simulink model "sistema_circuito2"  (R2025a)
settings: Solver=ode23tb  StartTime=0.0  StopTime=10.0  MaxStep=1E-3  RelTol=1e-3
libraries: fl_lib x12, ee_lib x3, nesl_utility x3
settings Model: Creator=Abigail VC  LastModifiedBy=Abigail VC
settings DataIOCC: TimeSaveName=t
settings DebuggingCC: AlgebraicLoopMsg=none  ArtificialAlgebraicLoopMsg=none  MaxConsecutiveZCsMsg=none

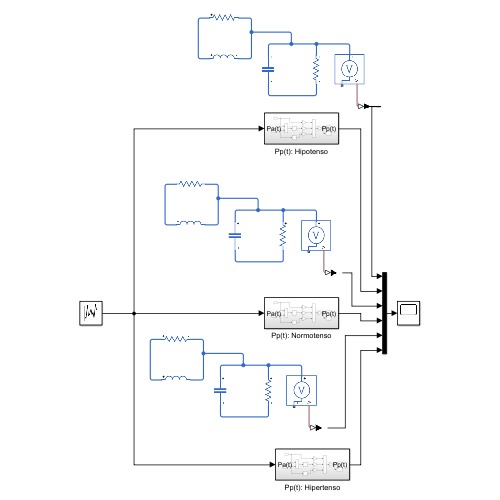
[thumbnail: Simulink's stored preview of the top-level diagram]
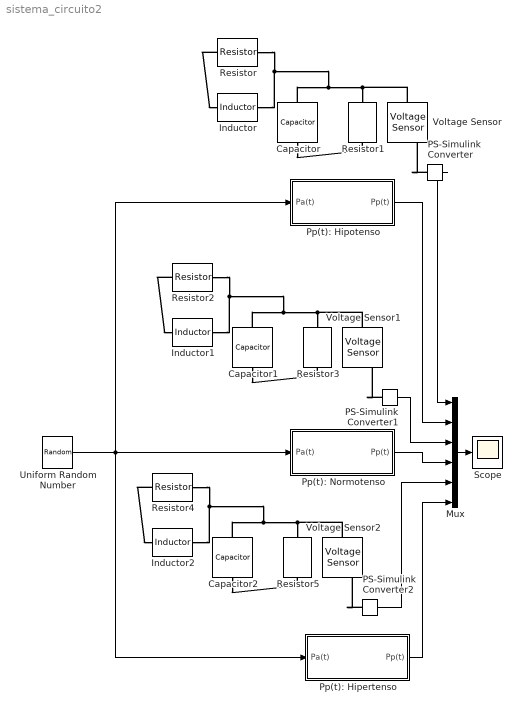
== system sistema_circuito2 ==
  Capacitor : fl_lib/Electrical/Electrical Elements/Capacitor  c=1e-6 F  r=1e-6 Ohm  g=0 1/Ohm  i_specify=off  i_priority=None  i=0 A  i_nominal_specify=off  i_nominal_value=1  i_nominal_unit=A  v_specify=off  v_priority=None  v=0 V  v_nominal_specify=off  v_nominal_value=1  v_nominal_unit=V  vc_specify=off  vc_priority=High  vc=0 V  vc_nominal_specify=off  vc_nominal_value=1  vc_nominal_unit=V
  Capacitor1 : fl_lib/Electrical/Electrical Elements/Capacitor  c=1e-6 F  r=1e-6 Ohm  g=0 1/Ohm  i_specify=off  i_priority=None  i=0 A  i_nominal_specify=off  i_nominal_value=1  i_nominal_unit=A  v_specify=off  v_priority=None  v=0 V  v_nominal_specify=off  v_nominal_value=1  v_nominal_unit=V  vc_specify=off  vc_priority=High  vc=0 V  vc_nominal_specify=off  vc_nominal_value=1  vc_nominal_unit=V
  Capacitor2 : fl_lib/Electrical/Electrical Elements/Capacitor  c=1e-6 F  r=1e-6 Ohm  g=0 1/Ohm  i_specify=off  i_priority=None  i=0 A  i_nominal_specify=off  i_nominal_value=1  i_nominal_unit=A  v_specify=off  v_priority=None  v=0 V  v_nominal_specify=off  v_nominal_value=1  v_nominal_unit=V  vc_specify=off  vc_priority=High  vc=0 V  vc_nominal_specify=off  vc_nominal_value=1  vc_nominal_unit=V
  Inductor : ee_lib/Passive/Inductor  l=1e-6 H  enable_L_tol=ee.enum.toleranceApplication.none  L_tol=20  tol_distribution=ee.enum.toleranceDistribution.uniform  nSigma=4  r=0 Ohm  g=1e-9 1/Ohm  enable_operating_limits=ee.enum.enable.no  operating_limit_action=ee.enum.passive.reportOpLim.warn  max_working_current=1 A  power_rating=1 W  i_L_specify=off  i_L_priority=High  i_L=0 A  i_L_nominal_specify=off  i_L_nominal_value=1  i_L_nominal_unit=A
  Inductor1 : ee_lib/Passive/Inductor  l=1e-6 H  enable_L_tol=ee.enum.toleranceApplication.none  L_tol=20  tol_distribution=ee.enum.toleranceDistribution.uniform  nSigma=4  r=0 Ohm  g=1e-9 1/Ohm  enable_operating_limits=ee.enum.enable.no  operating_limit_action=ee.enum.passive.reportOpLim.warn  max_working_current=1 A  power_rating=1 W  i_L_specify=off  i_L_priority=High  i_L=0 A  i_L_nominal_specify=off  i_L_nominal_value=1  i_L_nominal_unit=A
  Inductor2 : ee_lib/Passive/Inductor  l=1e-6 H  enable_L_tol=ee.enum.toleranceApplication.none  L_tol=20  tol_distribution=ee.enum.toleranceDistribution.uniform  nSigma=4  r=0 Ohm  g=1e-9 1/Ohm  enable_operating_limits=ee.enum.enable.no  operating_limit_action=ee.enum.passive.reportOpLim.warn  max_working_current=1 A  power_rating=1 W  i_L_specify=off  i_L_priority=High  i_L=0 A  i_L_nominal_specify=off  i_L_nominal_value=1  i_L_nominal_unit=A
  Mux : Mux  Inputs=6
  PS-Simulink Converter : nesl_utility/PS-Simulink Converter  PhysicalDomain=network_engine_domain  SubClassName=ps_output  LeftPortType=input  RightPortType=output  PseudoPeriodic=off  Frequencies=[]  VectorFormat=inherit  Unit=inherit  AffineConversion=off
  PS-Simulink Converter1 : nesl_utility/PS-Simulink Converter  PhysicalDomain=network_engine_domain  SubClassName=ps_output  LeftPortType=input  RightPortType=output  PseudoPeriodic=off  Frequencies=[]  VectorFormat=inherit  Unit=inherit  AffineConversion=off
  PS-Simulink Converter2 : nesl_utility/PS-Simulink Converter  PhysicalDomain=network_engine_domain  SubClassName=ps_output  LeftPortType=input  RightPortType=output  PseudoPeriodic=off  Frequencies=[]  VectorFormat=inherit  Unit=inherit  AffineConversion=off
  Pp(t): Hipertenso : Subsystem
  Pp(t): Hipotenso : Subsystem
  Pp(t): Normotenso : Subsystem
  Resistor{,1..5} (6 alike) : fl_lib/Electrical/Electrical Elements/Resistor  R=1 Ohm  i_specify=off  i_priority=None  i=0 A  i_nominal_specify=off  i_nominal_value=1  i_nominal_unit=A  v_specify=off  v_priority=None  v=0 V  v_nominal_specify=off  v_nominal_value=1  v_nominal_unit=V
  Scope : Scope
      settings: ActiveDisplayYMinimum=0.15751214924268458  ActiveDisplayYMaximum=0.91910296523276258
  Uniform Random Number : UniformRandomNumber  Minimum=-0.2  Seed=106  SampleTime=0.5
  Voltage Sensor : fl_lib/Electrical/Electrical Sensors/Voltage Sensor
  Voltage Sensor1 : fl_lib/Electrical/Electrical Sensors/Voltage Sensor
  Voltage Sensor2 : fl_lib/Electrical/Electrical Sensors/Voltage Sensor
  wires:
  Uniform Random Number/1 -> Pp(t): Normotenso/1(Pa(t)), Pp(t): Hipertenso/1(Pa(t)), Pp(t): Hipotenso/1(Pa(t))
  Pp(t): Hipotenso/1(Pp(t)) -> Mux/2
  Pp(t): Normotenso/1(Pp(t)) -> Mux/4
  Pp(t): Hipertenso/1(Pp(t)) -> Mux/6
  Mux/1 -> Scope/1
  PS-Simulink Converter/1 -> Mux/1
  PS-Simulink Converter1/1 -> Mux/3
  PS-Simulink Converter2/1 -> Mux/5
  connections:
  Resistor/LConn1 -- Inductor/LConn1
  Capacitor/LConn1 -- Resistor/RConn1 -- Inductor/RConn1 -- Voltage Sensor/LConn1 -- Resistor1/LConn1
  Capacitor/RConn1 -- Resistor1/RConn1
  PS-Simulink Converter/LConn1 -- Voltage Sensor/RConn1
  Resistor3/LConn1 -- Resistor2/RConn1 -- Inductor1/RConn1 -- Capacitor1/LConn1 -- Voltage Sensor1/LConn1
  PS-Simulink Converter1/LConn1 -- Voltage Sensor1/RConn1
  Capacitor1/RConn1 -- Resistor3/RConn1
  Resistor2/LConn1 -- Inductor1/LConn1
  Resistor5/LConn1 -- Resistor4/RConn1 -- Inductor2/RConn1 -- Capacitor2/LConn1 -- Voltage Sensor2/LConn1
  PS-Simulink Converter2/LConn1 -- Voltage Sensor2/RConn1
  Capacitor2/RConn1 -- Resistor5/RConn1
  Resistor4/LConn1 -- Inductor2/LConn1

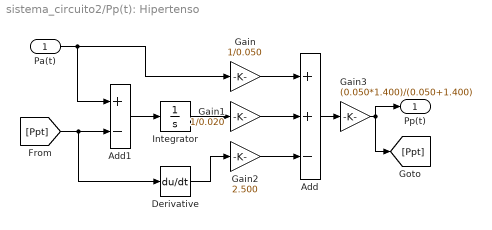
== system sistema_circuito2/Pp(t): Hipertenso ==
  Pa(t) : Inport
  Add : Sum  Inputs=++-
  Add1 : Sum  Inputs=+-
  Derivative : Derivative
  Gain : Gain  Gain=1/0.050
  Gain1 : Gain  Gain=1/0.020
  Gain2 : Gain  Gain=2.500
  Gain3 : Gain  Gain=(0.050*1.400)/(0.050+1.400)
  Integrator : Integrator
  Pp(t) : Outport
  wires:
  Pa(t)/1 -> Add1/1, Gain/1
  Gain/1 -> Add/1
  Integrator/1 -> Gain1/1
  Add1/1 -> Integrator/1
  [Ppt] -> Derivative/1, Add1/2
  Derivative/1 -> Gain2/1
  Gain1/1 -> Add/2
  Gain2/1 -> Add/3
  Add/1 -> Gain3/1
  Gain3/1 -> Pp(t)/1, [Ppt]

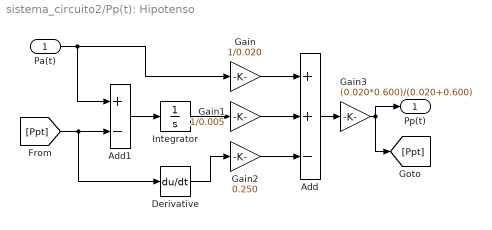
== system sistema_circuito2/Pp(t): Hipotenso ==
  Pa(t) : Inport
  Add : Sum  Inputs=++-
  Add1 : Sum  Inputs=+-
  Derivative : Derivative
  Gain : Gain  Gain=1/0.020
  Gain1 : Gain  Gain=1/0.005
  Gain2 : Gain  Gain=0.250
  Gain3 : Gain  Gain=(0.020*0.600)/(0.020+0.600)
  Integrator : Integrator
  Pp(t) : Outport
  wires:
  Pa(t)/1 -> Add1/1, Gain/1
  Gain/1 -> Add/1
  Integrator/1 -> Gain1/1
  Add1/1 -> Integrator/1
  [Ppt] -> Derivative/1, Add1/2
  Derivative/1 -> Gain2/1
  Gain1/1 -> Add/2
  Gain2/1 -> Add/3
  Add/1 -> Gain3/1
  Gain3/1 -> Pp(t)/1, [Ppt]

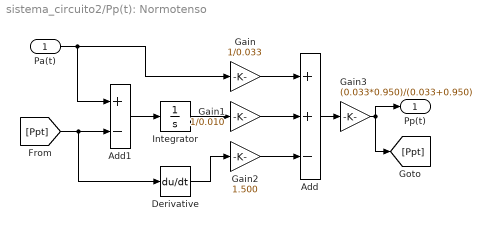
== system sistema_circuito2/Pp(t): Normotenso ==
  Pa(t) : Inport
  Add : Sum  Inputs=++-
  Add1 : Sum  Inputs=+-
  Derivative : Derivative
  Gain : Gain  Gain=1/0.033
  Gain1 : Gain  Gain=1/0.010
  Gain2 : Gain  Gain=1.500
  Gain3 : Gain  Gain=(0.033*0.950)/(0.033+0.950)
  Integrator : Integrator
  Pp(t) : Outport
  wires:
  Pa(t)/1 -> Add1/1, Gain/1
  Gain/1 -> Add/1
  Integrator/1 -> Gain1/1
  Add1/1 -> Integrator/1
  [Ppt] -> Derivative/1, Add1/2
  Derivative/1 -> Gain2/1
  Gain1/1 -> Add/2
  Gain2/1 -> Add/3
  Add/1 -> Gain3/1
  Gain3/1 -> Pp(t)/1, [Ppt]
